simulink model "medicalVentilatorSystemModel"  (R2022b)
settings: Solver=VariableStepAuto  StartTime=0.0  StopTime=30  RelTol=1e-3  AbsTol=1e-3
PreLoadFcn:
  | % medicalVentilatorSystemParams;
  | % controlParams;
  | % T_room=Hecate_T_room;
  | % T_body=Hecate_T_body;
InitFcn:
  | % T_room=Hecate_T_room;
  | % T_body=Hecate_T_body;
values from neighbouring files (symbols this model uses):
  cmH2O_to_Pa = 98.0665    [MVS.mat]    (also in medicalVentilatorSystemParams.m)
  D_trachea = 0.015    [MVS.mat]    (also in medicalVentilatorSystemParams.m)
  D_tube = 0.015    [MVS.mat]    (also in medicalVentilatorSystemParams.m)
  E_respiratory = 16    [MVS.mat]    (also in medicalVentilatorSystemParams.m)
  FRC = 2    [MVS.mat]    (also in medicalVentilatorSystemParams.m)
  L_trachea = 0.15    [MVS.mat]    (also in medicalVentilatorSystemParams.m)
  L_tube = 1    [MVS.mat]    (also in medicalVentilatorSystemParams.m)
  R_respiratory = 2    [MVS.mat]    (also in medicalVentilatorSystemParams.m)
  T_body = 37    [MVS.mat]    (also in medicalVentilatorSystemParams.m)
  T_humidifier = 40    [MVS.mat]    (also in medicalVentilatorSystemParams.m)
undefined symbols (not defined in the file or in its folder): Hecate_pressure, Hecate_T_body, Hecate_T_room, Hecate_tconst, Hecate_tconst2, Hecate_ttrans
libraries: fl_lib x74, nesl_utility x9, controlLibrary x1
(part 2 of 2)

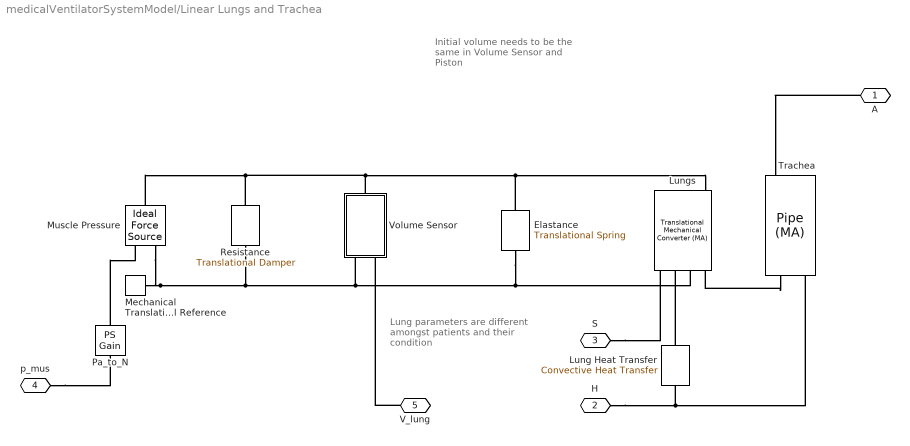
== system medicalVentilatorSystemModel/Linear Lungs and Trachea ==
  note: Lung parameters
      | are different
      | amongst patients
      | and their condition
  note: Initial volume needs
      | to be the same in
      | Volume Sensor
      | and Piston
  Elastance : fl_lib/Mechanical/Translational Elements/Translational Spring  spr_rate=E_respiratory*cmH2O_to_Pa/L_to_m3*A_interface^2 N/m  v_specify=off  v_priority=None  v=0 m/s  v_nominal_specify=off  v_nominal_unit=m/s  v_nominal_value=1  f_specify=off  f_priority=None  f=0 N  f_nominal_specify=off  f_nominal_unit=N  f_nominal_value=1  x_specify=on  x_priority=High  x=(vol_init - FRC)*L_to_m3/A_interface m  x_nominal_specify=off  x_nominal_unit=m  x_nominal_value=1
  Lung Heat Transfer : fl_lib/Thermal/Thermal Elements/Convective Heat Transfer  thermal_type=foundation.enum.constant_variable.constant  area=80 m^2  heat_tr_coeff=20 W/(m^2 * K)  min_heat_tr_coeff=1e-3 W/(K*m^2)  T_specify=off  T_priority=None  T=0 K  T_nominal_specify=off  T_nominal_unit=K  T_nominal_value=1  Q_specify=off  Q_priority=None  Q=0 W  Q_nominal_specify=off  Q_nominal_unit=W  Q_nominal_value=1
  Lungs : fl_lib/Moist Air/Elements/Translational Mechanical Converter (MA)  mech_orientation=simscape.enum.posneg.positive  displacement_spec=foundation.enum.DisplacementSpec.Calculate  length_init=vol_init* L_to_m3/A_interface m  interface_area=A_interface m^2  dead_volume=1e-6 m^3  area_A=pi*D_trachea^2/4 m^2  pressure_spec=foundation.enum.pressure_spec.atmospheric  environment_pressure=0.101325 MPa  RH_ws=1  time_constant=1e-3 s  moisture_trace_gas_source=foundation.enum.moisture_trace_gas_source.controlled  moisture_source_spec=foundation.enum.moisture_source_spec.vapor  moisture_mass_flow=0 kg/s  moisture_temperature_spec=foundation.enum.temperature_spec.atmospheric  moisture_temperature=293.15 K  trace_gas_mass_flow=0 kg/s  trace_gas_temperature_spec=foundation.enum.temperature_spec.atmospheric  trace_gas_temperature=293.15 K  p_I_specify=on  p_I_priority=High  p_I=0.101325 MPa  p_I_nominal_specify=off  p_I_nominal_unit=MPa  p_I_nominal_value=1  T_I_specify=on  T_I_priority=High  T_I=T_init degC  T_I_nominal_specify=off  T_I_nominal_unit=K  T_I_nominal_value=1  RH_I_specify=on  RH_I_priority=High  RH_I=1  RH_I_nominal_specify=off  RH_I_nominal_unit=1  RH_I_nominal_value=1  x_w_I_specify=off  x_w_I_priority=None  x_w_I=0  x_w_I_nominal_specify=off  x_w_I_nominal_unit=1  x_w_I_nominal_value=1  y_w_I_specify=off  y_w_I_priority=None  y_w_I=0  y_w_I_nominal_specify=off  y_w_I_nominal_unit=1  y_w_I_nominal_value=1  HR_I_specify=off  HR_I_priority=None  HR_I=0  HR_I_nominal_specify=off  HR_I_nominal_unit=1  HR_I_nominal_value=1  x_g_I_specify=on  x_g_I_priority=None  x_g_I=0  x_g_I_nominal_specify=off  x_g_I_nominal_unit=1  x_g_I_nominal_value=1  y_g_I_specify=on  y_g_I_priority=High  y_g_I=0.7  y_g_I_nominal_specify=off  y_g_I_nominal_unit=1  y_g_I_nominal_value=1
      settings: InternalSimscapePortConfiguration="{\"Bottom\":[],\"Left\":[{\"id\":\"A\",\"label\":\"A\",\"type\":\"foundation.moist_air.moist_air\"},{\"id\":\"C\",\"label\":\"C\",\"type\":\"foundation.mechanical.translational.translational\"},{\"id\":\"H\",\"label\":\"H\",\"type\":\"foundation.thermal.thermal\"},{\"id\":\"S\",\"label\":\"S\",\"type\":\"foundation.moist_air.moist_air_source\"}],\"Right\":[{\"id\":\"R\",\"label\":\"R\",\"type\":\"foundation.mechanical.translational.translational\"},{\"id\":\"W\",\"label\":\"W\",\"type\":\"output\"},{\"id\":\"F\",\"label\":\"F\",\"type\":\"output\"}],\"Top\":[]}"
  Mechanical Translational Reference : fl_lib/Mechanical/Translational Elements/Mechanical Translational Reference
  Muscle Pressure : fl_lib/Mechanical/Mechanical Sources/Ideal Force Source
  Pa_to_N : fl_lib/Physical Signals/Functions/PS Gain  gain=A_interface N/Pa
  Resistance : fl_lib/Mechanical/Translational Elements/Translational Damper  D=(R_respiratory * cmH2O_to_Pa/ L_to_m3)*A_interface^2 N/(m/s)  v_specify=off  v_priority=None  v=0 m/s  v_nominal_specify=off  v_nominal_unit=m/s  v_nominal_value=1  f_specify=off  f_priority=None  f=0 N  f_nominal_specify=off  f_nominal_unit=N  f_nominal_value=1
  Trachea : fl_lib/Moist Air/Elements/Pipe (MA)  length=L_trachea m  area=pi*D_trachea^2/4 m^2  Dh=D_trachea m  length_add=0.1 m  roughness=15e-6 m  Re_lam=2000  Re_tur=4000  shape_factor=64  Nu_lam=3.66  wall_condensation=simscape.enum.onoff.off  RH_ws=1  time_constant=1e-3 s  moisture_trace_gas_source=foundation.enum.moisture_trace_gas_source.none  moisture_source_spec=foundation.enum.moisture_source_spec.vapor  moisture_mass_flow=0 kg/s  moisture_temperature_spec=foundation.enum.temperature_spec.atmospheric  moisture_temperature=293.15 K  trace_gas_mass_flow=0 kg/s  trace_gas_temperature_spec=foundation.enum.temperature_spec.atmospheric  trace_gas_temperature=293.15 K  p_I_specify=on  p_I_priority=High  p_I=0.101325 MPa  p_I_nominal_specify=off  p_I_nominal_unit=MPa  p_I_nominal_value=1  T_I_specify=on  T_I_priority=High  T_I=T_init degC  T_I_nominal_specify=off  T_I_nominal_unit=K  T_I_nominal_value=1  RH_I_specify=on  RH_I_priority=High  RH_I=1  RH_I_nominal_specify=off  RH_I_nominal_unit=1  RH_I_nominal_value=1  x_w_I_specify=off  x_w_I_priority=None  x_w_I=0  x_w_I_nominal_specify=off  x_w_I_nominal_unit=1  x_w_I_nominal_value=1  y_w_I_specify=off  y_w_I_priority=None  y_w_I=0  y_w_I_nominal_specify=off  y_w_I_nominal_unit=1  y_w_I_nominal_value=1  HR_I_specify=off  HR_I_priority=None  HR_I=0  HR_I_nominal_specify=off  HR_I_nominal_unit=1  HR_I_nominal_value=1  x_g_I_specify=on  x_g_I_priority=None  x_g_I=0  x_g_I_nominal_specify=off  x_g_I_nominal_unit=1  x_g_I_nominal_value=1  y_g_I_specify=on  y_g_I_priority=High  y_g_I=0.7  y_g_I_nominal_specify=off  y_g_I_nominal_unit=1  y_g_I_nominal_value=1
  Volume Sensor : Subsystem  mask(Volume Data){vol_init=vol_init}
      mask prompts: vol_init "Initial lung volume [L]"
      mask help: This subsystem reports the lung volume. Because the Interface cross-sectional area parameter in the lung model is set to 1 m^2, therefore 1 m of measured displacement is equivalent to 1 m^3 of lung volume and 1 N of measured force is equivalent to 1 Pa of pressure.
      mask init:
      | L_to_m3 = 1e-3;
  A : PMIOPort  Side=Right
  H : PMIOPort  Port=2  Side=Left
  S : PMIOPort  Port=3  Side=Left
  p_mus : PMIOPort  Port=4  Side=Left
  V_lung : PMIOPort  Port=5  Side=Right
  connections:
  Pa_to_N/RConn1 -- Muscle Pressure/RConn1
  p_mus/RConn1 -- Pa_to_N/LConn1
  V_lung/RConn1 -- Volume Sensor/RConn2
  S/RConn1 -- Lungs/LConn4
  A/RConn1 -- Trachea/RConn1
  Lungs/LConn2 -- Volume Sensor/RConn1 -- Resistance/RConn1 -- Muscle Pressure/RConn2 -- Mechanical Translational Reference/LConn1 -- Elastance/RConn1
  Lung Heat Transfer/LConn1 -- Lungs/LConn3
  Trachea/LConn2 -- Lung Heat Transfer/RConn1 -- H/RConn1
  Lungs/RConn1 -- Resistance/LConn1 -- Muscle Pressure/LConn1 -- Volume Sensor/LConn1 -- Elastance/LConn1
  Trachea/LConn1 -- Lungs/LConn1

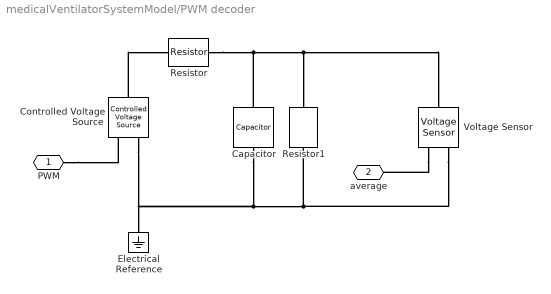
== system medicalVentilatorSystemModel/PWM decoder ==
  Capacitor : fl_lib/Electrical/Electrical Elements/Capacitor  c=47 uF  r=1e-6 Ohm  g=0 1/Ohm  i_specify=off  i_priority=None  i=0 A  i_nominal_specify=off  i_nominal_unit=A  i_nominal_value=1  v_specify=off  v_priority=None  v=0 V  v_nominal_specify=off  v_nominal_unit=V  v_nominal_value=1  vc_specify=off  vc_priority=High  vc=0 V  vc_nominal_specify=off  vc_nominal_unit=V  vc_nominal_value=1
  Controlled Voltage Source : fl_lib/Electrical/Electrical Sources/Controlled Voltage Source
  Electrical Reference : fl_lib/Electrical/Electrical Elements/Electrical Reference
  Resistor : fl_lib/Electrical/Electrical Elements/Resistor  R=1 kOhm  i_specify=off  i_priority=None  i=0 A  i_nominal_specify=off  i_nominal_unit=A  i_nominal_value=1  v_specify=off  v_priority=None  v=0 V  v_nominal_specify=off  v_nominal_unit=V  v_nominal_value=1
  Resistor1 : fl_lib/Electrical/Electrical Elements/Resistor  R=100 kOhm  i_specify=off  i_priority=None  i=0 A  i_nominal_specify=off  i_nominal_unit=A  i_nominal_value=1  v_specify=off  v_priority=None  v=0 V  v_nominal_specify=off  v_nominal_unit=V  v_nominal_value=1
  Voltage Sensor : fl_lib/Electrical/Electrical Sensors/Voltage Sensor
  PWM : PMIOPort  Side=Left
  average : PMIOPort  Port=2  Side=Right
  connections:
  PWM/RConn1 -- Controlled Voltage Source/RConn1
  Resistor/RConn1 -- Capacitor/LConn1 -- Resistor1/LConn1 -- Voltage Sensor/LConn1
  Controlled Voltage Source/LConn1 -- Resistor/LConn1
  Voltage Sensor/RConn2 -- Resistor1/RConn1 -- Capacitor/RConn1 -- Electrical Reference/LConn1 -- Controlled Voltage Source/RConn2
  Voltage Sensor/RConn1 -- average/RConn1

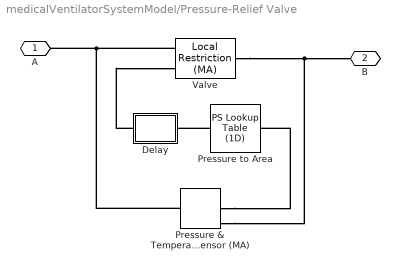
== system medicalVentilatorSystemModel/Pressure-Relief Valve ==
  Delay : Subsystem  mask{tau=tau, x0=A_leak}
      mask prompts: tau "Time constant (s)"; x0 "Initial output"
  Pressure & Temperature Sensor (MA) : fl_lib/Moist Air/Sensors/Pressure & Temperature Sensor (MA)
      settings: InternalSimscapePortConfiguration="{\"Bottom\":[],\"Left\":[{\"id\":\"A\",\"label\":\"A\",\"type\":\"foundation.moist_air.moist_air\"}],\"Right\":[{\"id\":\"B\",\"label\":\"B\",\"type\":\"foundation.moist_air.moist_air\"},{\"id\":\"P\",\"label\":\"P\",\"type\":\"output\"},{\"id\":\"T\",\"label\":\"T\",\"type\":\"output\"}],\"Top\":[]}"
  Pressure to Area : fl_lib/Physical Signals/Lookup Tables/PS Lookup Table (1D)  x=[0 p_set p_max p_max+1] Pa  f=[A_leak, A_leak, A_max, A_max] m^2  interp_method=simscape.enum.interpolation.linear  extrap_method=simscape.enum.extrapolation.nearest
  Valve : fl_lib/Moist Air/Elements/Local Restriction (MA)  restriction_type=foundation.enum.restriction_type.variable  restriction_area=0.001 m^2  min_area=A_leak/2 m^2  max_area=(A_max + A_port)/2 m^2  area=A_port m^2  Cd=Cd  B_lam=0.999
  A : PMIOPort  Side=Left
  B : PMIOPort  Port=2  Side=Right
  connections:
  Pressure & Temperature Sensor (MA)/LConn1 -- A/RConn1 -- Valve/LConn1
  Pressure & Temperature Sensor (MA)/RConn1 -- B/RConn1 -- Valve/RConn1
  Pressure & Temperature Sensor (MA)/RConn2 -- Pressure to Area/LConn1
  Pressure to Area/RConn1 -- Delay/LConn1
  Delay/RConn1 -- Valve/LConn2

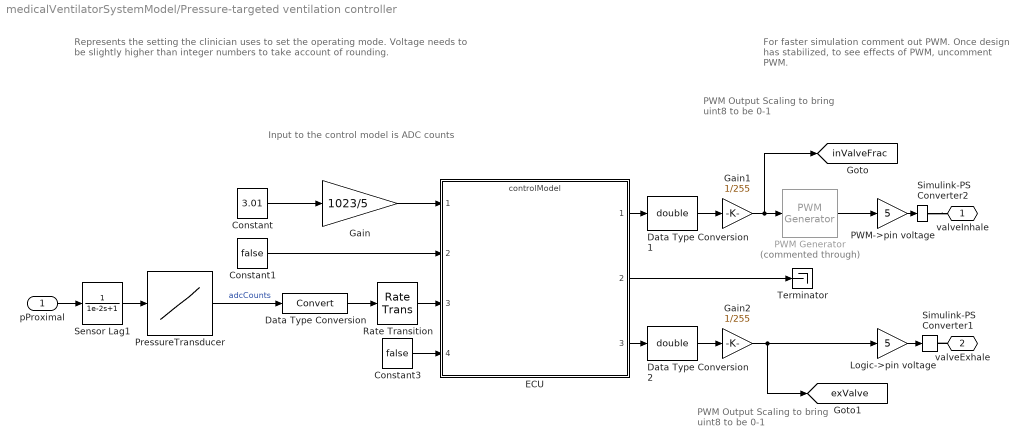
== system medicalVentilatorSystemModel/Pressure-targeted ventilation controller ==
  note: For faster simulation comment out PWM.
      | Once design has stabilized, to see effects
      | of PWM, uncomment PWM.
  note: PWM Output
      | Scaling to bring
      | uint8 to be 0-1
  note: Input to the control model is ADC counts
  note: Represents the setting the clinician uses to set the operating mode.
      | Voltage needs to be slightly higher than integer numbers to take
      | account of rounding.
  note: PWM Output
      | Scaling to bring
      | uint8 to be 0-1
  pProximal : Inport
  Constant : Constant  Value=3.01
  Constant1 : Constant  Value=false
  Constant3 : Constant  Value=false
  Data Type Conversion : DataTypeConversion  RndMeth=Floor
  Data Type Conversion1 : DataTypeConversion  OutDataTypeStr=double  SaturateOnIntegerOverflow=off  RndMeth=Floor
  Data Type Conversion2 : DataTypeConversion  OutDataTypeStr=double  SaturateOnIntegerOverflow=off  RndMeth=Floor
  ECU : ModelReference  ModelNameDialog=controlModel  SimulationMode=Normal  ModelReferenceVersion=6.0
  Gain : Gain  Gain=1023/5  OutDataTypeStr=uint16
  Gain1 : Gain  Gain=1/255
  Gain2 : Gain  Gain=1/255
  Logic->pin voltage : Gain  Gain=5
  PWM Generator : controlLibrary/PWM Generator  Commented=through  CarrCount=Up  Tper=0.001/0.05  Ts=0.001
  PWM->pin voltage : Gain  Gain=5
  PressureTransducer : Lookup_n-D  NumberOfTableDimensions=1  BreakpointsForDimension1=[0 50]  BreakpointsForDimension1DataTypeStr=double  Table=[0.5 4.5]*1023/5  TableDataTypeStr=Inherit: Inherit from 'Table data'  ExtrapMethod=Clip  InternalRulePriority=Speed  OutDataTypeStr=Inherit: Inherit via back propagation  RndMeth=Simplest
  Rate Transition : RateTransition  OutPortSampleTime=0.01
  Sensor Lag1 : TransferFcn  Denominator=[1e-2 1]
  Simulink-PS Converter1 : nesl_utility/Simulink-PS Converter  PhysicalDomain=network_engine_domain  SubClassName=ps_input  LeftPortType=input  RightPortType=output  PseudoPeriodic=off  Frequencies=[]  NoiseDistribution=none  NoiseParameters=[]  Unit=V  AffineConversion=off  FilteringAndDerivatives=provide  SimscapeFilterOrder=1  InputFilterTimeConstant=0.001  UdotUserProvided=0
  Simulink-PS Converter2 : nesl_utility/Simulink-PS Converter  PhysicalDomain=network_engine_domain  SubClassName=ps_input  LeftPortType=input  RightPortType=output  PseudoPeriodic=off  Frequencies=[]  NoiseDistribution=none  NoiseParameters=[]  Unit=V  AffineConversion=off  FilteringAndDerivatives=provide  SimscapeFilterOrder=1  InputFilterTimeConstant=0.001  UdotUserProvided=0
  Terminator : Terminator
  valveInhale : PMIOPort  Side=Right
  valveExhale : PMIOPort  Port=2  Side=Right
  tag scope: exValve=global, inValveFrac=global
  wires:
  PWM->pin voltage/1 -> Simulink-PS Converter2/1
  Constant1/1 -> ECU/2
  Constant/1 -> Gain/1
  Constant3/1 -> ECU/4
  ECU/2 -> Terminator/1
  pProximal/1 -> Sensor Lag1/1
  PressureTransducer/1 -> Data Type Conversion/1  "adcCounts"
  Gain/1 -> ECU/1
  Data Type Conversion/1 -> Rate Transition/1
  Logic->pin voltage/1 -> Simulink-PS Converter1/1
  Sensor Lag1/1 -> PressureTransducer/1
  ECU/3 -> Data Type Conversion2/1
  ECU/1 -> Data Type Conversion1/1
  Rate Transition/1 -> ECU/3
  Data Type Conversion1/1 -> Gain1/1
  Data Type Conversion2/1 -> Gain2/1
  Gain1/1 -> [inValveFrac], PWM Generator/1
  Gain2/1 -> Logic->pin voltage/1, [exValve]
  PWM Generator/1 -> PWM->pin voltage/1
  connections:
  Simulink-PS Converter2/RConn1 -- valveInhale/RConn1
  valveExhale/RConn1 -- Simulink-PS Converter1/RConn1

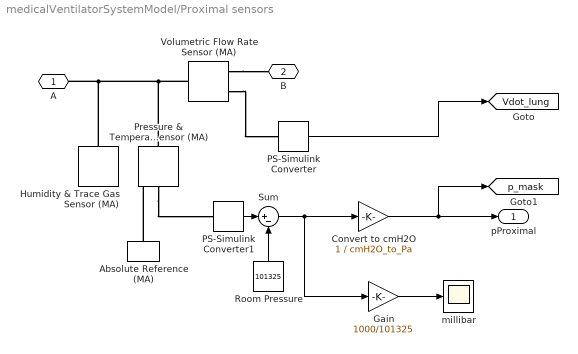
== system medicalVentilatorSystemModel/Proximal sensors ==
  Absolute Reference (MA) : fl_lib/Moist Air/Elements/Absolute Reference (MA)
  Convert to cmH2O : Gain  Gain=1 / cmH2O_to_Pa
  Gain : Gain  Gain=1000/101325
  Humidity & Trace Gas Sensor (MA) : fl_lib/Moist Air/Sensors/Humidity & Trace Gas Sensor (MA)  moisture_spec=foundation.enum.moisture_spec.relative_humidity  trace_gas_spec=foundation.enum.trace_gas_spec.mass_fraction
      settings: InternalSimscapePortConfiguration="{\"Bottom\":[],\"Left\":[{\"id\":\"A\",\"label\":\"A\",\"type\":\"foundation.moist_air.moist_air\"}],\"Right\":[{\"id\":\"W\",\"label\":\"W\",\"type\":\"output\"},{\"id\":\"G\",\"label\":\"G\",\"type\":\"output\"}],\"Top\":[]}"
  PS-Simulink Converter : nesl_utility/PS-Simulink Converter  PhysicalDomain=network_engine_domain  SubClassName=ps_output  LeftPortType=input  RightPortType=output  PseudoPeriodic=off  Frequencies=[]  VectorFormat=1-D array  Unit=l/min  AffineConversion=off
  PS-Simulink Converter1 : nesl_utility/PS-Simulink Converter  PhysicalDomain=network_engine_domain  SubClassName=ps_output  LeftPortType=input  RightPortType=output  PseudoPeriodic=off  Frequencies=[]  VectorFormat=1-D array  Unit=Pa  AffineConversion=off
  Pressure & Temperature Sensor (MA) : fl_lib/Moist Air/Sensors/Pressure & Temperature Sensor (MA)
      settings: InternalSimscapePortConfiguration="{\"Bottom\":[],\"Left\":[{\"id\":\"A\",\"label\":\"A\",\"type\":\"foundation.moist_air.moist_air\"}],\"Right\":[{\"id\":\"B\",\"label\":\"B\",\"type\":\"foundation.moist_air.moist_air\"},{\"id\":\"P\",\"label\":\"P\",\"type\":\"output\"},{\"id\":\"T\",\"label\":\"T\",\"type\":\"output\"}],\"Top\":[]}"
  Room Pressure : Constant  Value=101325
  Sum : Sum  Inputs=|+-
  Volumetric Flow Rate Sensor (MA) : fl_lib/Moist Air/Sensors/Volumetric Flow Rate Sensor (MA)  volumetric_flow_conditions=foundation.enum.volumetric_flow_conditions.actual  p_std=0.101325 MPa  T_std=20 degC  RH_std=0.65
      settings: InternalSimscapePortConfiguration="{\"Bottom\":[],\"Left\":[{\"id\":\"A\",\"label\":\"A\",\"type\":\"foundation.moist_air.moist_air\"}],\"Right\":[{\"id\":\"B\",\"label\":\"B\",\"type\":\"foundation.moist_air.moist_air\"},{\"id\":\"V\",\"label\":\"V\",\"type\":\"output\"}],\"Top\":[]}"
  millibar : Scope
  A : PMIOPort  Side=Right
  B : PMIOPort  Port=2  Side=Left
  pProximal : Outport
  tag scope: Vdot_lung=global, p_mask=global
  wires:
  PS-Simulink Converter/1 -> [Vdot_lung]
  Convert to cmH2O/1 -> [p_mask], pProximal/1
  PS-Simulink Converter1/1 -> Sum/1
  Sum/1 -> Gain/1, Convert to cmH2O/1
  Room Pressure/1 -> Sum/2
  Gain/1 -> millibar/1
  connections:
  Volumetric Flow Rate Sensor (MA)/LConn1 -- Pressure & Temperature Sensor (MA)/LConn1 -- Humidity & Trace Gas Sensor (MA)/LConn1 -- A/RConn1
  Volumetric Flow Rate Sensor (MA)/RConn1 -- B/RConn1
  Volumetric Flow Rate Sensor (MA)/RConn2 -- PS-Simulink Converter/LConn1
  Absolute Reference (MA)/LConn1 -- Pressure & Temperature Sensor (MA)/RConn1
  Pressure & Temperature Sensor (MA)/RConn2 -- PS-Simulink Converter1/LConn1

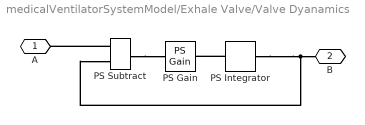
== system medicalVentilatorSystemModel/Exhale Valve/Valve Dyanamics ==
  PS Gain : fl_lib/Physical Signals/Functions/PS Gain  gain=1/tau 1/s
  PS Integrator : fl_lib/Physical Signals/Linear Operators/PS Integrator  reset_method=foundation.enum.IntegratorResetSpec.None  initial_condition_spec=foundation.enum.IntegratorICSpec.Internal  saturation_spec=foundation.enum.IntegratorSaturationSpec.None  saturation_source_spec=foundation.enum.IntegratorSaturationSourceSpec.Internal  x0=x0 in^2  xu=inf s  xl=-inf s
  PS Subtract : fl_lib/Physical Signals/Functions/PS Subtract
  A : PMIOPort  Side=Left
  B : PMIOPort  Port=2  Side=Right
  connections:
  PS Integrator/LConn1 -- PS Gain/RConn1
  PS Subtract/LConn1 -- A/RConn1
  PS Subtract/RConn1 -- PS Gain/LConn1
  B/RConn1 -- PS Subtract/LConn2 -- PS Integrator/RConn1

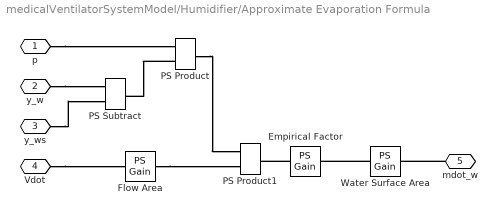
== system medicalVentilatorSystemModel/Humidifier/Approximate Evaporation Formula ==
  Empirical Factor : fl_lib/Physical Signals/Functions/PS Gain  gain=5e-8 kg/J
  Flow Area : fl_lib/Physical Signals/Functions/PS Gain  gain=1 / (pi*D_tube^2/4) 1/m^2
  PS Product : fl_lib/Physical Signals/Functions/PS Product
  PS Product1 : fl_lib/Physical Signals/Functions/PS Product
  PS Subtract : fl_lib/Physical Signals/Functions/PS Subtract
  Water Surface Area : fl_lib/Physical Signals/Functions/PS Gain  gain=A_humidifier m^2
  p : PMIOPort  Side=Left
  y_w : PMIOPort  Port=2  Side=Left
  y_ws : PMIOPort  Port=3  Side=Left
  Vdot : PMIOPort  Port=4  Side=Left
  mdot_w : PMIOPort  Port=5  Side=Right
  connections:
  y_w/RConn1 -- PS Subtract/LConn2
  y_ws/RConn1 -- PS Subtract/LConn1
  p/RConn1 -- PS Product/LConn1
  PS Product/LConn2 -- PS Subtract/RConn1
  PS Product/RConn1 -- PS Product1/LConn1
  Flow Area/RConn1 -- PS Product1/LConn2
  Empirical Factor/LConn1 -- PS Product1/RConn1
  Water Surface Area/LConn1 -- Empirical Factor/RConn1
  mdot_w/RConn1 -- Water Surface Area/RConn1
  Vdot/RConn1 -- Flow Area/LConn1

== system medicalVentilatorSystemModel/Inhale Valve/Valve Dyanamics ==
  PS Gain : fl_lib/Physical Signals/Functions/PS Gain  gain=1/tau 1/s
  PS Integrator : fl_lib/Physical Signals/Linear Operators/PS Integrator  reset_method=foundation.enum.IntegratorResetSpec.None  initial_condition_spec=foundation.enum.IntegratorICSpec.Internal  saturation_spec=foundation.enum.IntegratorSaturationSpec.None  saturation_source_spec=foundation.enum.IntegratorSaturationSourceSpec.Internal  x0=x0 in^2  xu=inf s  xl=-inf s
  PS Subtract : fl_lib/Physical Signals/Functions/PS Subtract
  A : PMIOPort  Side=Left
  B : PMIOPort  Port=2  Side=Right
  connections:
  PS Integrator/RConn1 -- PS Subtract/LConn2 -- B/RConn1
  PS Subtract/RConn1 -- PS Gain/LConn1
  PS Subtract/LConn1 -- A/RConn1
  PS Integrator/LConn1 -- PS Gain/RConn1

== system medicalVentilatorSystemModel/Linear Lungs and Trachea/Volume Sensor ==
  Ideal Translational Motion Sensor : fl_lib/Mechanical/Mechanical Sensors/Ideal Translational Motion Sensor  reference=foundation.enum.MeasurementReference.difference  acceleration_port=false  velocity_port=true  position_port=true  offset=vol_init*L_to_m3/A_interface m
  pos_to_vol : fl_lib/Physical Signals/Functions/PS Gain  gain=A_interface m^2
  R : PMIOPort  Side=Left
  C : PMIOPort  Port=2  Side=Right
  V_lung : PMIOPort  Port=3  Side=Right
  connections:
  V_lung/RConn1 -- pos_to_vol/RConn1
  Ideal Translational Motion Sensor/RConn3 -- pos_to_vol/LConn1
  Ideal Translational Motion Sensor/RConn1 -- C/RConn1
  Ideal Translational Motion Sensor/LConn1 -- R/RConn1

== system medicalVentilatorSystemModel/Pressure-Relief Valve/Delay ==
  PS Gain : fl_lib/Physical Signals/Functions/PS Gain  gain=1/tau 1/s
  PS Integrator : fl_lib/Physical Signals/Linear Operators/PS Integrator  reset_method=foundation.enum.IntegratorResetSpec.None  initial_condition_spec=foundation.enum.IntegratorICSpec.Internal  saturation_spec=foundation.enum.IntegratorSaturationSpec.None  saturation_source_spec=foundation.enum.IntegratorSaturationSourceSpec.Internal  x0=x0 m^2  xu=inf s  xl=-inf s
  PS Subtract : fl_lib/Physical Signals/Functions/PS Subtract
  A : PMIOPort  Side=Left
  B : PMIOPort  Port=2  Side=Right
  connections:
  PS Integrator/RConn1 -- PS Subtract/LConn2 -- B/RConn1
  PS Subtract/RConn1 -- PS Gain/LConn1
  PS Subtract/LConn1 -- A/RConn1
  PS Integrator/LConn1 -- PS Gain/RConn1

== stateflow chart medicalVentilatorSystemModel/Test Assessment ==
  state step_1
    state step_1_1
      verify(pressure<=30);
      verify(volume <=6 && volume >= 0);
    state step_1_2
    (default) -> (junction 22)
    step_1 -> (junction 22)
    (junction 22) -> (junction 23) [order 1] : [t < 30
        | ]
    (junction 23) -> step_1_1 [order 1] : [~in(step_1.step_1_1)]
    (junction 22) -> (junction 31) [order 2]
    (junction 23) -> (junction 26) [order 2]
    (junction 31) -> (junction 32)
    (junction 32) -> step_1_2 [order 1] : [~in(step_1.step_1_2)]
    (junction 32) -> (junction 35) [order 2]
  (default) -> step_1
  data: pressure input; volume input

== stateflow chart medicalVentilatorSystemModel/FitnessConverter_Hecate ==
  state step_1
    fitness_1 = Inf;
    fitness_2 = Inf;
    state step_1_1
      fitness_1 = 30-(pressure);
      fitness_2 = min([6-(volume);volume-(0);]);
    state step_1_2
      fitness_1 = Inf;
      fitness_2 = Inf;
    (default) -> (junction 4)
    step_1_2 -> (junction 4) : [(t < 30)]
    (junction 4) -> step_1_1 [order 1] : [t < 30]
    (junction 4) -> step_1_2 [order 2] : []
    step_1_1 -> (junction 4) : [~(t < 30)]
  (default) -> step_1
  data: pressure input; volume input; fitness_1 output; fitness_2 output

== stateflow chart medicalVentilatorSystemModel/Test Sequence ==
  state MVS_square
    state step_1
      muscle_pressure=0;
      T_body=Hecate_T_body;
      T_room=Hecate_T_room;
      %temperature = 37 + 3/30*ramp(et);
    state step_2
      muscle_pressure=Hecate_pressure;
      T_body=Hecate_T_body;
      T_room=Hecate_T_room;
    state step_3
      muscle_pressure=0;
    (default) -> MVS_square.step_1
    MVS_square.step_1 -> MVS_square.step_2 : [
        | after(10,sec)
        | ]
    MVS_square.step_2 -> MVS_square.step_3 : [
        | after(20,sec)
        | ]
    MVS_square.step_3 -> MVS_square.step_2 : [
        | after(2,sec)
        | ]
  state MVS_trapezoid
    state step_1
      muscle_pressure=0;
      T_body=Hecate_T_body;
      T_room=Hecate_T_room;
      %temperature = 37 + 3/30*ramp(et);
    state step_2
      muscle_pressure=(Hecate_pressure/0.25)*(t-10);
      %muscle_pressure = ramp(t-10)*Hecate_pressure/0.25;
    state step_3
      muscle_pressure=Hecate_pressure;
      T_body=Hecate_T_body;
      T_room=Hecate_T_room;
    state step_4
      muscle_pressure=-(Hecate_pressure/0.25)*(t-11.75)+Hecate_pressure;
      %muscle_pressure = -ramp(t-11.75)*Hecate_pressure/0.25 + Hecate_pressure;
    state step_5_DELAY
      muscle_pressure=0;
    state step_6
      muscle_pressure=(Hecate_pressure/0.25)*(t-14);
      %muscle_pressure = ramp(t-10)*Hecate_pressure/0.25;
    state step_7
      muscle_pressure=Hecate_pressure;
    state step_8
      muscle_pressure=-(Hecate_pressure/0.25)*(t-15.75)+Hecate_pressure;
    state step_9
      muscle_pressure=0;
    (default) -> MVS_trapezoid.step_1
    MVS_trapezoid.step_1 -> MVS_trapezoid.step_2 : [
        | after(10,sec)
        | ]
    MVS_trapezoid.step_2 -> MVS_trapezoid.step_3 : [
        | after(0.25,sec)
        | ]
    MVS_trapezoid.step_3 -> MVS_trapezoid.step_4 : [
        | after(1.5,sec)
        | ]
    MVS_trapezoid.step_4 -> step_5_DELAY : [
        | after(0.25,sec)
        | ]
    step_5_DELAY -> step_6 : [
        | after(2,sec)
        | ]
    step_6 -> step_7 : [
        | after(0.25,sec)
        | ]
    step_7 -> step_8 : [
        | after(1.5,sec)
        | ]
    step_8 -> step_9 : [
        | after(0.25,sec)
        | ]
  state MVS_trapezoid_rep
    state step_1
      muscle_pressure = Hecate_pressure*2*t/Hecate_ttrans;
      T_body=Hecate_T_body;
      T_room=Hecate_T_room;
    state step_2
      muscle_pressure = Hecate_pressure;
    state step_3
      muscle_pressure = Hecate_pressure - Hecate_pressure*(2*et/Hecate_ttrans);
    state step_4
      muscle_pressure = -Hecate_pressure;
    state step_5
      muscle_pressure = -Hecate_pressure + Hecate_pressure*(2*et/Hecate_ttrans);
    (default) -> MVS_trapezoid_rep.step_1
    MVS_trapezoid_rep.step_1 -> MVS_trapezoid_rep.step_2 : [
        | et >=Hecate_ttrans/2
        | ]
    (junction 145) -> MVS_trapezoid_rep.step_2
    (junction 154) -> (junction 145)
    MVS_trapezoid_rep.step_2 -> MVS_trapezoid_rep.step_3 : [
        | et >= Hecate_tconst
        | ]
    MVS_trapezoid_rep.step_3 -> MVS_trapezoid_rep.step_4 : [
        | et >= Hecate_ttrans
        | ]
    MVS_trapezoid_rep.step_4 -> step_5 : [
        | et >= Hecate_tconst
        | ]
    step_5 -> (junction 154) : [
        | et >= Hecate_ttrans
        | ]
  state MVS_square_rep
    state step_1
      muscle_pressure  = 0;
      T_body=Hecate_T_body;
      T_room=Hecate_T_room;
    state step_2
      muscle_pressure = Hecate_pressure*square(et/Hecate_tconst);
    state step_3
      muscle_pressure = Hecate_pressure*square(et/Hecate_tconst2);
    (default) -> MVS_square_rep.step_1
    MVS_square_rep.step_1 -> MVS_square_rep.step_2 : [
        | after(10,sec)
        | ]
    MVS_square_rep.step_2 -> MVS_square_rep.step_3 : [
        | after(10,sec)
        | ]
  (default) -> MVS_square [order 1] : [Active_Scenario_Index == 1]
  (default) -> MVS_trapezoid [order 2] : [Active_Scenario_Index == 2]
  (default) -> MVS_trapezoid_rep [order 3] : [Active_Scenario_Index == 3]
  (default) -> MVS_square_rep [order 4] : {assert(Active_Scenario_Index == 4,'The value of Scenario Parameter ''Active_Scenario_Index'' is not valid. Use the index of the scenario to specify it.')}
  data: Hecate_pressure parameter; T_room output; T_body output; muscle_pressure output; Hecate_T_body parameter; Hecate_T_room parameter; Active_Scenario_Index parameter =1; Hecate_ttrans parameter; Hecate_tconst parameter; Hecate_tconst2 parameter
